simulink model "Astatizm1"  (R2017a)
settings: Solver=VariableStepAuto  StartTime=0.0  StopTime=30  MaxStep=0.10001  MinStep=0.1  RelTol=1e-6
undefined symbols (not defined in the file): a, k
settings Model: Creator=User  LastModifiedBy=User

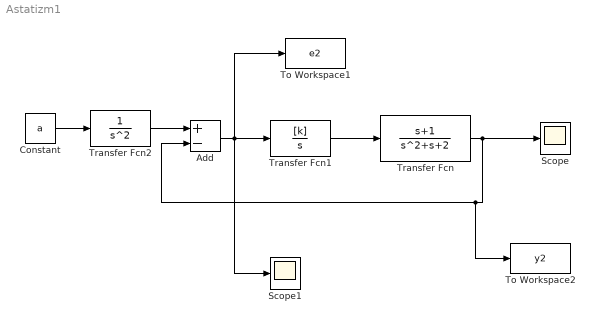
== system Astatizm1 ==
  Add : Sum  Inputs=+-
  Constant : Constant  Value=a
  Scope : Scope
  Scope1 : Scope
  To Workspace1 : ToWorkspace  VariableName=e2  SampleTime=-1
  To Workspace2 : ToWorkspace  VariableName=y2  SampleTime=-1
  Transfer Fcn : TransferFcn  Numerator=[1 1]  Denominator=[1 1 2]
  Transfer Fcn1 : TransferFcn  Numerator=[k]  Denominator=[1 0]
  Transfer Fcn2 : TransferFcn  Denominator=[1 0 0]
  wires:
  Add/1 -> Transfer Fcn1/1, To Workspace1/1, Scope1/1
  Transfer Fcn/1 -> To Workspace2/1, Add/2, Scope/1
  Constant/1 -> Transfer Fcn2/1
  Transfer Fcn1/1 -> Transfer Fcn/1
  Transfer Fcn2/1 -> Add/1
